simulink model "Euler_Example"  (R2024b)
settings: Solver=VariableStepAuto  StartTime=0.0  StopTime=10.0  RelTol=1e-3
settings Model: Creator=user  LastModifiedBy=user

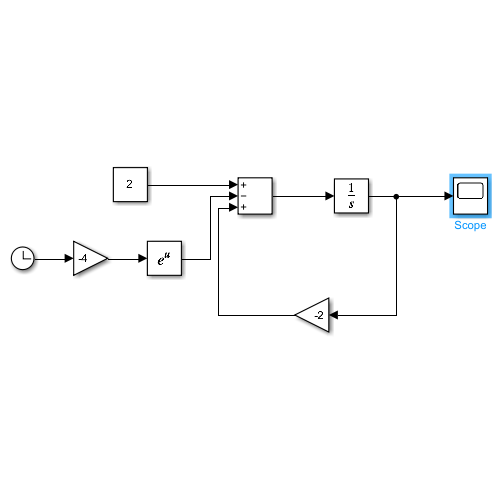
[thumbnail: Simulink's stored preview of the top-level diagram]
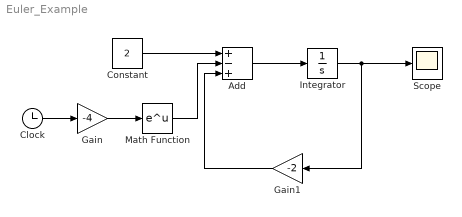
== system Euler_Example ==
  Add : Sum  Inputs=+-+
  Clock : Clock
  Constant : Constant  Value=2
  Gain : Gain  Gain=-4
  Gain1 : Gain  Gain=-2
  Integrator : Integrator  InitialCondition=1
  Math Function : Math
  Scope : Scope
  wires:
  Constant/1 -> Add/1
  Clock/1 -> Gain/1
  Gain/1 -> Math Function/1
  Math Function/1 -> Add/2
  Add/1 -> Integrator/1
  Integrator/1 -> Scope/1, Gain1/1
  Gain1/1 -> Add/3
